simulink model "task2_Hbridge_dc_dc_converter"  (R2025b)
settings: Solver=FixedStepDiscrete  StartTime=0.0  StopTime=0.005  FixedStep=5e-7  RelTol=1e-3
libraries: dspstat3 x2, simulink x2
settings Model: Creator=Администратор  LastModifiedBy=Администратор

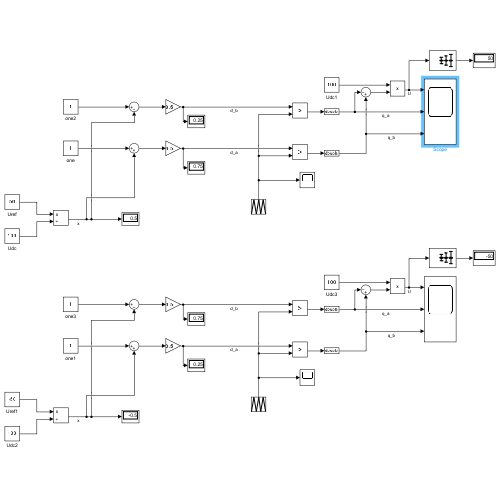
[thumbnail: Simulink's stored preview of the top-level diagram]
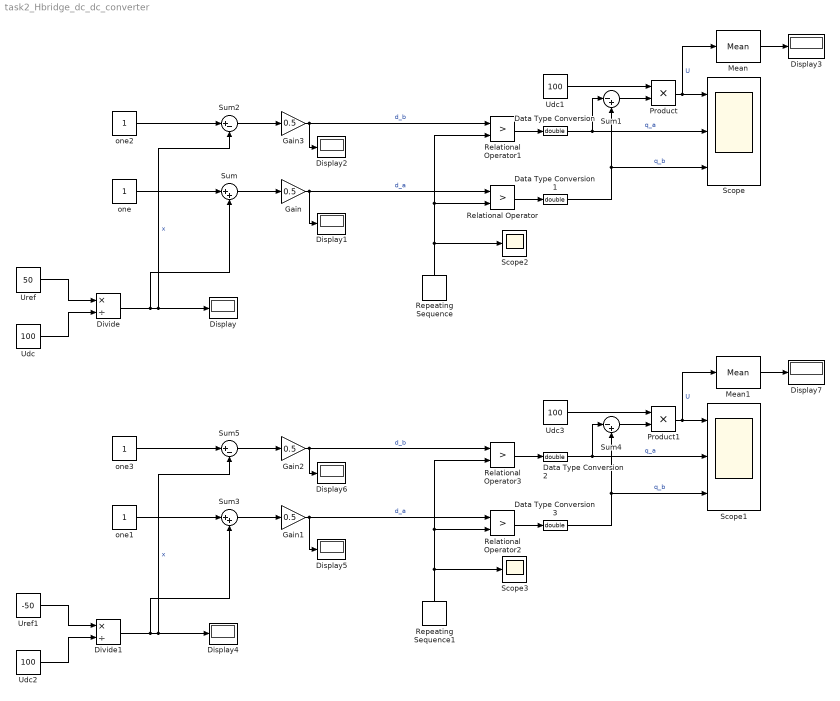
== system task2_Hbridge_dc_dc_converter ==
  Data Type Conversion{,1..3} (4 alike) : DataTypeConversion  OutDataTypeStr=double  SaturateOnIntegerOverflow=off  RndMeth=Floor
  Display{,1..7} (8 alike) : Display
  Divide : Product  Inputs=*/
  Divide1 : Product  Inputs=*/
  Gain{,1..3} (4 alike) : Gain  Gain=0.5
  Mean : dspstat3/Mean  run=on  reset_popup=None  directionMode=Each column  dimension=1  roiEnable=off  roiType=Rectangles  roiPortion=Entire ROI  roiOutput=Individual statistics for each ROI  roiFlag=off  roundingMode=Floor  overflowMode=off  outputDataTypeStr=Inherit: Same as accumulator  outputMin=[]  outputMax=[]  outputLastDataTypeStr=Inherit: Same as accumulator
  Mean1 : dspstat3/Mean  run=on  reset_popup=None  directionMode=Each column  dimension=1  roiEnable=off  roiType=Rectangles  roiPortion=Entire ROI  roiOutput=Individual statistics for each ROI  roiFlag=off  roundingMode=Floor  overflowMode=off  outputDataTypeStr=Inherit: Same as accumulator  outputMin=[]  outputMax=[]  outputLastDataTypeStr=Inherit: Same as accumulator
  Product : Product
  Product1 : Product
  Relational Operator{,1..3} (4 alike) : RelationalOperator  Operator=>  OutDataTypeStr=boolean  RndMeth=Simplest  InputSameDT=off
  Repeating Sequence : simulink/Sources/Repeating Sequence  rep_seq_t=[0 25e-6 50e-6]  rep_seq_y=[0 1 0]
  Repeating Sequence1 : simulink/Sources/Repeating Sequence  rep_seq_t=[0 25e-6 50e-6]  rep_seq_y=[0 1 0]
  Scope : Scope  NumInputPorts=3
      settings: ActiveDisplayString=3  ActiveDisplayYMinimum=-0.12499999999999997  ActiveDisplayYMaximum=1.125
  Scope1 : Scope  NumInputPorts=3
      settings: ActiveDisplayString=3  ActiveDisplayYMinimum=-0.12499999999999997  ActiveDisplayYMaximum=1.125
  Scope2 : Scope
      settings: ActiveDisplayYMinimum=0.1271576523322262  ActiveDisplayYMaximum=0.36965917517358116  DataLoggingVariableName=ScopeData2
  Scope3 : Scope
      settings: ActiveDisplayYMinimum=0.1271576523322262  ActiveDisplayYMaximum=0.36965917517358116  DataLoggingVariableName=ScopeData3
  Sum : Sum  Inputs=|++
  Sum1 : Sum  Inputs=|-+
  Sum2 : Sum  Inputs=|+-
  Sum3 : Sum  Inputs=|++
  Sum4 : Sum  Inputs=|-+
  Sum5 : Sum  Inputs=|+-
  Udc{,1..3} (4 alike) : Constant  Value=100
  Uref : Constant  Value=50
  Uref1 : Constant  Value=-50
  one{,1..3} (4 alike) : Constant
  wires:
  Uref/1 -> Divide/1
  Udc/1 -> Divide/2
  Divide/1 -> Sum2/2, Display/1, Sum/2  "x"
  one/1 -> Sum/1
  Sum/1 -> Gain/1
  Gain/1 -> Relational Operator/1, Display1/1  "d_a"
  Gain3/1 -> Relational Operator1/1, Display2/1  "d_b"
  Sum2/1 -> Gain3/1
  one2/1 -> Sum2/1
  Relational Operator/1 -> Data Type Conversion1/1
  Relational Operator1/1 -> Data Type Conversion/1
  Product/1 -> Scope/1, Mean/1  "U"
  Repeating Sequence/1 -> Relational Operator/2, Relational Operator1/2, Scope2/1
  Mean/1 -> Display3/1
  Data Type Conversion/1 -> Sum1/1, Scope/2  "q_a"
  Data Type Conversion1/1 -> Sum1/2, Scope/3  "q_b"
  Sum1/1 -> Product/2
  Udc1/1 -> Product/1
  Udc3/1 -> Product1/1
  Sum4/1 -> Product1/2
  Data Type Conversion3/1 -> Scope1/3, Sum4/2  "q_b"
  Data Type Conversion2/1 -> Scope1/2, Sum4/1  "q_a"
  Mean1/1 -> Display7/1
  Repeating Sequence1/1 -> Scope3/1, Relational Operator3/2, Relational Operator2/2
  Product1/1 -> Mean1/1, Scope1/1  "U"
  Relational Operator3/1 -> Data Type Conversion2/1
  Relational Operator2/1 -> Data Type Conversion3/1
  one3/1 -> Sum5/1
  Sum5/1 -> Gain2/1
  Gain2/1 -> Display6/1, Relational Operator3/1  "d_b"
  Gain1/1 -> Display5/1, Relational Operator2/1  "d_a"
  Sum3/1 -> Gain1/1
  one1/1 -> Sum3/1
  Divide1/1 -> Sum3/2, Display4/1, Sum5/2  "x"
  Udc2/1 -> Divide1/2
  Uref1/1 -> Divide1/1
